simulink model "SIMUR10E"  (R2025a)
settings: Solver=FixedStepAuto  StartTime=0.0  StopTime=200  RelTol=1e-3
libraries: ros2lib x3, instrumentseriallib x2, sldrtlib x1
settings Model: Creator=piete  LastModifiedBy=po
settings OptimizationCC: DefaultParameterBehavior=Inlined  EnhancedBackFolding=on  PassReuseOutputArgsAs=Individual arguments  ZeroExternalMemoryAtStartup=off  ZeroInternalMemoryAtStartup=off  MaxStackSize=64  OptimizeBlockOrder=speed  DifferentSizesBufferReuse=on  OptimizationCustomize=off  EfficientTunableParamExpr=on
settings DebuggingCC: ParameterTunabilityLossMsg=error
settings RTWCC: SystemTargetFile=ert.tlc  HardwareBoard=Robot Operating System 2 (ROS 2)  TLCOptions="-aInlineSetEventsForThisBaseRateFcn=TLC_FALSE -aSuppressMultiTaskScheduler=TLC_FALSE  -aRateBasedStepFcn=0"  TemplateMakefile=ert_default_tmf  Toolchain=Colcon Tools  TargetLang=C++  Description=Embedded Coder
settings CodeAppCC: ForceParamTrailComments=on  IgnoreCustomStorageClasses=off  OperatorAnnotations=on  SimulinkDataObjDesc=on  SFDataObjDesc=on  InsertBlockDesc=on
settings ERTTargetCC: ExtModeTransport=2.0  ExtModeAutomaticAllocSize=off  RootIOFormat=Structure reference  CodeInterfacePackaging=C++ class  SupportVariableSizeSignals=on

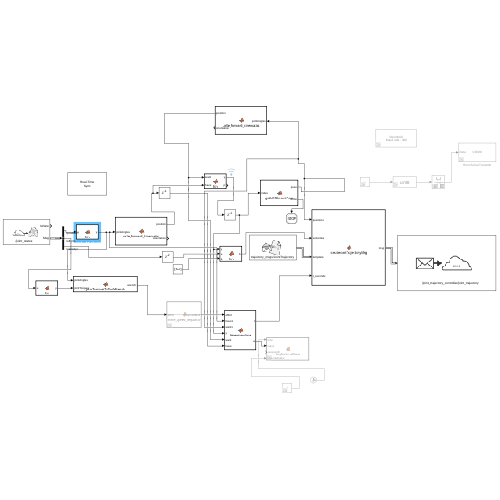
[thumbnail: Simulink's stored preview of the top-level diagram]
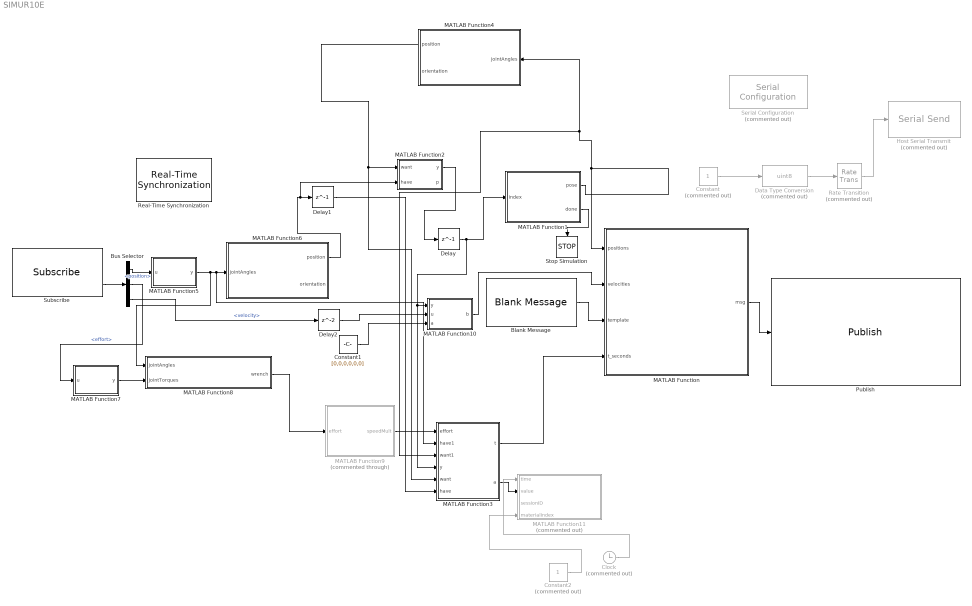
== system SIMUR10E ==
  Blank Message : ros2lib/Blank Message  messageClass=Message  entityType=trajectory_msgs/JointTrajectory  messageType=trajectory_msgs/JointTrajectory  SampleTime=inf
  Bus Selector : BusSelector  OutputSignals=position,effort,velocity
  Clock : Clock  Commented=on
  Constant : Constant  Commented=on
  Constant1 : Constant  Value=[0,0,0,0,0,0]
  Constant2 : Constant  Commented=on
  Data Type Conversion : DataTypeConversion  Commented=on  OutDataTypeStr=uint8  SaturateOnIntegerOverflow=off  RndMeth=Floor
  Delay : Delay  DelayLength=1  InitialCondition=1
  Delay1 : Delay  DelayLength=1  InitialCondition=0  InputProcessing=Columns as channels (frame based)
  Delay2 : Delay
  Host Serial Transmit : instrumentseriallib/Serial Send  Commented=on  PortSel=COM8  Port=COM8  ComPort=COM8  Header='S'  Terminator=Custom terminator  CustomTerminator='E'  EnableBlockingMode=off  SimulateUsing=Interpreted execution  BlockInModel=on  aMode=5
      settings: LibrarySourceBlock=mcblib/Protection and Diagnostics/Host Serial Transmit
  MATLAB Function : MATLAB Function  TreatAsAtomicUnit=on
  MATLAB Function1 : MATLAB Function  TreatAsAtomicUnit=on
  MATLAB Function10 : MATLAB Function  TreatAsAtomicUnit=on
  MATLAB Function11 : MATLAB Function  Commented=on  TreatAsAtomicUnit=on
  MATLAB Function2 : MATLAB Function  TreatAsAtomicUnit=on
  MATLAB Function3 : MATLAB Function  TreatAsAtomicUnit=on
  MATLAB Function4 : MATLAB Function  TreatAsAtomicUnit=on
  MATLAB Function5 : MATLAB Function  TreatAsAtomicUnit=on
  MATLAB Function6 : MATLAB Function  TreatAsAtomicUnit=on
  MATLAB Function7 : MATLAB Function  TreatAsAtomicUnit=on
  MATLAB Function8 : MATLAB Function  TreatAsAtomicUnit=on
  MATLAB Function9 : MATLAB Function  Commented=through  TreatAsAtomicUnit=on
  Publish : ros2lib/Publish  topicSource=Select from ROS network  topic=/joint_trajectory_controller/joint_trajectory  messageType=trajectory_msgs/JointTrajectory  QOSHistory=Keep last  QOSDepth=10  QOSReliability=Reliable  QOSDurability=Volatile  QOSDeadline=Inf  QOSLifespan=Inf  QOSLiveliness=Automatic  QOSLeaseDuration=Inf  QOSAvoidROSNamespaceConventions=off
  Rate Transition : RateTransition  Commented=on  OutPortSampleTime=2
  Real-Time Synchronization : sldrtlib/Real-Time Synchronization  SampleTime=0.001  MaxMissedTicks=100000000000000000000000000000000000  ShowMissedTicks=off  YieldWhenWaiting=off
  Serial Configuration : instrumentseriallib/Serial Configuration  Priority=-200000  Commented=on  PortSel=/dev/ttyS0  Port=/dev/ttyS0  ComPort=/dev/ttyS0  BaudRate=300  DataBits=8  Parity=none  StopBits=1  ByteOrder=little-endian  FlowControl=none  Timeout=10  SimulateUsing=Interpreted execution  BlockInModel=on  aMode=1
      settings: LibrarySourceBlock=c2000lib/Host Communication/Serial Configuration
  Stop Simulation : Stop
  Subscribe : ros2lib/Subscribe  topicSource=Select from ROS network  topic=/joint_states  messageType=sensor_msgs/JointState  sampleTime=-1  QOSHistory=Keep last  QOSDepth=10  QOSReliability=Reliable  QOSDurability=Volatile  QOSDeadline=Inf  QOSLifespan=Inf  QOSLiveliness=Automatic  QOSLeaseDuration=Inf  QOSAvoidROSNamespaceConventions=off
  wires:
  Subscribe/2 -> Bus Selector/1
  Blank Message/1 -> MATLAB Function/3(template)
  MATLAB Function5/1(y) -> MATLAB Function8/1(jointAngles), MATLAB Function3/2(have1), MATLAB Function6/1(jointAngles)
  Bus Selector/1 -> MATLAB Function5/1(u)  "<position>"
  MATLAB Function7/1(y) -> MATLAB Function8/2(jointTorques)
  Bus Selector/2 -> MATLAB Function7/1(u)  "<effort>"
  MATLAB Function1/2(done) -> Stop Simulation/1
  MATLAB Function/1(msg) -> Publish/1
  MATLAB Function1/1(pose) -> MATLAB Function/1(positions), MATLAB Function4/1(jointAngles), MATLAB Function3/3(want1)
  MATLAB Function8/1(wrench) -> MATLAB Function9/1(effort)
  MATLAB Function9/1(speedMult) -> MATLAB Function3/1(effort)
  Constant/1 -> Data Type Conversion/1
  Data Type Conversion/1 -> Rate Transition/1
  Rate Transition/1 -> Host Serial Transmit/1
  MATLAB Function3/1(t) -> MATLAB Function/4(t_seconds)
  MATLAB Function6/1(position) -> MATLAB Function2/2(have), Delay1/1
  Delay1/1 -> MATLAB Function3/6(have)
  MATLAB Function4/1(position) -> MATLAB Function3/5(want), MATLAB Function2/1(want)
  MATLAB Function10/1(b) -> MATLAB Function/2(velocities)
  Bus Selector/3 -> Delay2/1  "<velocity>"
  Delay2/1 -> MATLAB Function10/2(u)
  Constant1/1 -> MATLAB Function10/3(a)
  MATLAB Function3/2(a) -> MATLAB Function11/2(value)
  Clock/1 -> MATLAB Function11/1(time)
  Constant2/1 -> MATLAB Function11/4(materialIndex)
  MATLAB Function2/1(y) -> Delay/1
  Delay/1 -> MATLAB Function3/4(y), MATLAB Function10/1(y), MATLAB Function1/1(index)

== matlab function SIMUR10E/MATLAB Function11 ==
  data: time input; value input; sessionID input; materialIndex input
function logMaterialData(time, value, sessionID, materialIndex)
%#codegen

persistent dataLog

% Define material names based on index
materialList = ["Steel", "Aluminum", "Plastic"];
materialID = materialList(materialIndex);

% Initialize if empty
if isempty(dataLog)
    dataLog = repmat(struct(), 10, 1); % Up to 10 sessions
end

% Convert struct field manually
sessionField = sessionID;
materialField = materialIndex;

% Preallocate if needed
if ~isfield(dataLog(sessionField), "Time")
    dataLog(sessionField).Time = cell(length(materialList), 1);
    dataLog(sessionField).Value = cell(length(materialList), 1);
end

% Append
if isempty(dataLog(sessionField).Time{materialField})
    dataLog(sessionField).Time{materialField} = time;
    dataLog(sessionField).Value{materialField} = value;
else
    dataLog(sessionField).Time{materialField}(end+1, 1) = time;
    dataLog(sessionField).Value{materialField}(end+1, :) = value;
end

% Export to base workspace after each step (optional)
coder.extrinsic('assignin');
assignin('base', 'dataLog', dataLog);

== matlab function SIMUR10E/MATLAB Function1 ==
  data: index input; pose output; done output
function [pose, done] = getUR10eJointPose(index)
% Returns a 1x6 joint pose vector and a "done" flag

coder.extrinsic('warning');

persistent angles
coder.varsize('angles', [Inf, 6], [1 0]);

if isempty(angles)
    data = coder.load('ur10e_joint_poses.mat');
    if isfield(data, 'validAngles') && size(data.validAngles, 2) == 6
        angles = data.validAngles;
    else
        angles = zeros(1, 6);
        warning('Invalid or missing validAngles in MAT file');
    end
end

n = size(angles, 1);
index = max(1, min(index, n));
pose = angles(index, :);

if isempty(pose)
    pose = zeros(1, 6);
end

% Done when we reached the last pose
done = (index >= n);
end

== matlab function SIMUR10E/MATLAB Function ==
  data: positions input; velocities input; msg output Bus: SL_Bus_trajectory_msgs_JointTrajectory; template input; t_seconds input
function msg = createJointTrajectoryMsg(positions, velocities, template, t_seconds)
msg = template;

joint_names = {'shoulder_pan_joint', 'shoulder_lift_joint', ...
               'elbow_joint', 'wrist_1_joint', ...
               'wrist_2_joint', 'wrist_3_joint'};

for i = 1:6
    name_uint8 = uint8(joint_names{i});
    msg.joint_names(i).data = zeros(128,1,'uint8');
    msg.joint_names(i).data(1:numel(name_uint8)) = name_uint8(:);
    msg.joint_names(i).data_SL_Info.CurrentLength = uint32(numel(name_uint8));
end
msg.joint_names_SL_Info.CurrentLength = uint32(6);

pt = msg.points(1);
pt.positions = zeros(128,1);
pt.positions(1:6) = positions(:);
pt.positions_SL_Info.CurrentLength = uint32(6);

pt.velocities = zeros(128,1);
pt.velocities(1:6) = velocities(:);
pt.velocities_SL_Info.CurrentLength = uint32(6);

pt.accelerations = zeros(128,1);
pt.accelerations_SL_Info.CurrentLength = uint32(0);
pt.effort = zeros(128,1);
pt.effort_SL_Info.CurrentLength = uint32(0);

% Properly set time_from_start
% For example, time_from_start = 100.0000001 seconds

pt.time_from_start.sec = int32(floor(t_seconds));        % 100 seconds
pt.time_from_start.nanosec = uint32(round(5)); % 100 nanoseconds


msg.points(1) = pt;
msg.points_SL_Info.CurrentLength = uint32(1);

msg.header.stamp.sec = int32(0);
msg.header.stamp.nanosec = uint32(0);
msg.header.frame_id = zeros(128,1,'uint8');
msg.header.frame_id_SL_Info.CurrentLength = uint32(0);
end

== matlab function SIMUR10E/MATLAB Function2 ==
  data: want input; y output; have input; p output
function [y,p]= fcn(want, have)
persistent step
if isempty(step)
    step = 1;
end

% Compute position error
po = zeros(1,3);
for n = 1:3
    po(1,n) = (have(1,n) - want(1,n));  % Circular indexing
end
p=sqrt(po(1,1)^2+po(1,2)^2+po(1,3)^2);
% Check if close enough to desired position
if p <= 0.00001
    step = step + 1;
end

y = step;

== matlab function SIMUR10E/MATLAB Function3 ==
  data: effort input; have1 input; want1 input; y input; want input; have input; t output; a output
function [t,a]= determinetime(effort, have1, want1, y, want, have)
% if y==1
%     b=3;
% else
%     b=0;
% end
% data = load('toolpath_info.mat');
% toolpath_length = data.toolpath_length;
% toolpath_num_points = data.toolpath_num_points;
% tt=toolpath_length/toolpath_num_points;
po = zeros(1,3);
for n = 1:3
    po(1,n) = (have(1,n) - want(1,n));  % Circular indexing
end
p=sqrt(po(1,1)^2+po(1,2)^2+po(1,3)^2);
ab= abs(effort);
a=sqrt(ab(1)^2+ab(2)^2+ab(3)^2);
hawa=zeros(1,6);
if y==1
    for i=1:6
  hawa(i)=abs(have1(i)-want1(i));
    end
    t=max(hawa)*8;
else
t=p*(a*3)^10;
end
% t=p*00+p*a^2*10;

end

== matlab function SIMUR10E/MATLAB Function4 ==
  data: jointAngles input; position output; orientation output
function [position, orientation] = ur3e_forward_kinematics(jointAngles)
%#codegen

% Inputs:
% jointAngles - 1x6 array [rad] of UR3e joint angles
% Outputs:
% position - 1x3 [m] XYZ position of tool tip
% orientation - 1x4 quaternion [qx qy qz qw] of tool tip

% Load robot model once and persist in memory
persistent robot toolTransform
if isempty(robot)
    robot = loadrobot('universalUR3e', 'DataFormat', 'row');
    
    % Define tool transform (211 mm link + 4.5 mm tool radius)
    toolOffset = trvec2tform([0 0 -0.29418]);  % in meters
    toolRotation = axang2tform([1 0 0 pi]);    % flip around X
    toolTransform = toolRotation * toolOffset;
end

% Compute forward kinematics to 'tool0'
tform = getTransform(robot, jointAngles, 'tool0');

% Apply tool transform
fullTform = tform * toolTransform;

% Extract position and orientation
position = fullTform(1:3, 4)';
rotm = fullTform(1:3, 1:3);
orientation = rotm2quat(rotm);  % [qx qy qz qw]
end

== matlab function SIMUR10E/MATLAB Function5 ==
  data: u input; y output
function y = fcn(u)
y=zeros(1,6);
b = u(1:6)';
y(1)=b(3);
y(2)=b(2);
y(3)=b(1);
y(4)=b(4);
y(5)=b(5);
y(6)=b(6);

== matlab function SIMUR10E/MATLAB Function6 ==
  data: jointAngles input; position output; orientation output
function [position, orientation] = ur3e_forward_kinematics(jointAngles)
%#codegen

% Inputs:
% jointAngles - 1x6 array [rad] of UR3e joint angles
% Outputs:
% position - 1x3 [m] XYZ position of tool tip
% orientation - 1x4 quaternion [qx qy qz qw] of tool tip

% Load robot model once and persist in memory
persistent robot toolTransform
if isempty(robot)
    robot = loadrobot('universalUR3e', 'DataFormat', 'row');
    
    % Define tool transform (211 mm link + 4.5 mm tool radius)
    toolOffset = trvec2tform([0 0 -0.29418]);  % in meters
    toolRotation = axang2tform([1 0 0 pi]);    % flip around X
    toolTransform = toolRotation * toolOffset;
end

% Compute forward kinematics to 'tool0'
tform = getTransform(robot, jointAngles, 'tool0');

% Apply tool transform
fullTform = tform * toolTransform;

% Extract position and orientation
position = fullTform(1:3, 4)';
rotm = fullTform(1:3, 1:3);
orientation = rotm2quat(rotm);  % [qx qy qz qw]
end

== matlab function SIMUR10E/MATLAB Function7 ==
  data: u input; y output
function y = fcn(u)
y=zeros(1,6);
b = u(1:6)';
y(1)=b(3);
y(2)=b(2);
y(3)=b(1);
y(4)=b(4);
y(5)=b(5);
y(6)=b(6);

== matlab function SIMUR10E/MATLAB Function8 ==
  data: jointAngles input; wrench output; jointTorques input
function wrench = jointTorquesToToolWrench(jointAngles, jointTorques)
%#codegen
% Inputs:
% jointAngles  - 1x6 vector of UR3e joint positions [rad]
% jointTorques - 1x6 vector of joint torques [Nm]
% Output:
% wrench - 1x6 vector [Fx Fy Fz Mx My Mz] in N and N·m

persistent robot
if isempty(robot)
    robot = loadrobot('universalUR3e', 'DataFormat', 'row');
end

% Compute geometric Jacobian at current config
J = geometricJacobian(robot, jointAngles, 'tool0');

% Solve J' * wrench = torques  → wrench = pinv(J') * torques
wrench = (pinv(J')) * jointTorques(:);
%wrench = wrench;  % return as row vector
end

== matlab function SIMUR10E/MATLAB Function9 ==
  data: effort input; speedMult output
function speedMult = force_speed_regulator(effort)
%#codegen
currentForce=sqrt(effort(1)^2+effort(2)^2+effort(3)^2);
% Persistent variable to store previous force value
persistent prevForce
if isempty(prevForce)
    prevForce = currentForce;  % Initialize on first run
end

% Parameters
deadband = 3.5;         % Sensor noise threshold
desiredForce = 20;      % Target force in N (can be set as parameter)
k = 0.02;               % Proportional gain
maxMult = 1.5;
minMult = 0.5;

% Compute force trend
deltaForce = currentForce - prevForce;

% Apply deadband filtering
if abs(deltaForce) < deadband
    deltaForce = 0;
end

% Compute force error
forceError = desiredForce - currentForce;

% Compute speed multiplier
speedMult = 1 + k * forceError;

% Clamp speed multiplier to [0.5, 1.5]
speedMult = max(min(speedMult, maxMult), minMult);

% Update previous force for next time step
prevForce = currentForce;

== matlab function SIMUR10E/MATLAB Function10 ==
  data: y input; u input; b output; a input
function b = fcn(y, u, a)
b = zeros(1, 6); % Fixed-size initialization
if y == 1
    b(:) = u(1:6); % Ensure assignment maintains size
else
    b(:) = a(1:6); % Explicitly maintain size
end
